simulink model "hexacopter_sim"  (R2024b)
settings: Solver=VariableStepAuto  StartTime=0  StopTime=100  FixedStep=0.1  RelTol=1e-3  EnableMultiTasking=on
values from neighbouring files (symbols this model uses):
  A = [zeros(4), eye(4); zeros(4),zeros(4)]    [hexacopter_par.m]
  b = 1.177*10^-5    (= 1.177e-05)    [hexacopter_par.m]
  B = [zeros(4) ... (first row only)    [hexacopter_par.m]
  C_obs = eye(8)    [hexacopter_par.m]
  d = 1.855*10^-7    (= 1.855e-07)    [hexacopter_par.m]
  fault_level = 0    [hexacopter_par.m]
  g = 9.81    [hexacopter_par.m]
  Ic = Ic + temp    [hexacopter_par.m]
  Ix = Ic(1,1)    [hexacopter_par.m]
  Iy = Ic(2,2)    [hexacopter_par.m]
  Iz = Ic(3,3)    [hexacopter_par.m]
  J_T = 1/2 *m_r* R_r^2    (= 0.0001)    [hexacopter_par.m]
  K_lqr = lqr(A', C_obs', Q, R)'    [hexacopter_par.m]
  K_phi = 0.03    [hexacopter_par.m]
  K_psi = 0.1    [hexacopter_par.m]
  K_theta = 0.03    [hexacopter_par.m]
  Kx = .1    (= 0.1)    [hexacopter_par.m]
  Ky = .1    (= 0.1)    [hexacopter_par.m]
  Kz = .1    (= 0.1)    [hexacopter_par.m]
  L = 0.275    [hexacopter_par.m]
  m = 2.5    [hexacopter_par.m]
  M_RB = [ m*eye(3) , zeros(3) ; zeros(3) , Ic ]    [hexacopter_par.m]
  motor_index = 3    [hexacopter_par.m]
  T_psinv = pinv(T)    [hexacopter_par.m]
libraries: slpidlib x19, simulink_extras x17, aerolibutil x2, matrix_library x2, vrlib x2, slctrl_smc x1
(part 1 of 3)
settings Model: Creator=The MathWorks, Inc.  LastModifiedBy=edtob
settings SolverCC: AlgebraicLoopSolver=TrustRegion
settings DataIOCC: LimitDataPoints=on  SaveFormat=Array  SaveOutput=off  SignalLogging=off  DSMLogging=off  SaveTime=off  ReturnWorkspaceOutputs=off
settings OptimizationCC: BlockReduction=off  BufferReuse=off  LifeSpan=inf
settings DebuggingCC: AlgebraicLoopMsg=none  ParameterPrecisionLossMsg=none  AllowSymbolicDim=off  PregeneratedLibrarySubsystemCodeDiagnostic=none  SFUnexpectedBacktrackingDiag=warning  SFNoUnconditionalDefaultTransitionDiag=warning  SFExecutionAtInitializationDiag=none  ArithmeticOperatorsInVariantConditions=warning
settings HardwareCC: ProdBitPerPointer=32  ProdBitPerSizeT=32  ProdBitPerPtrDiffT=32  ProdLargestAtomicFloat=None  ProdIntDivRoundTo=Undefined  ProdEndianess=Unspecified  ProdWordSize=32  ProdHWDeviceType=32-bit Generic
settings ModelReferenceCC: EnableRefExpFcnMdlSchedulingChecks=on  PropagateSignalLabelsOutOfModel=off
settings SFSimCC: SimUseLocalCustomCode=off  CustomCodeUndefinedFunction=UseInterfaceOnly
settings RTWCC: RTWUseLocalCustomCode=off  GPUComputeCapability=3.5  DLArmComputeVersion=19.05
settings CodeAppCC: StateflowObjectComments=on
settings GRTTargetCC: TargetLangStandard=C89/C90 (ANSI)
settings ConfigComp: CovMetricSettings=dw  CovSaveCumulativeToWorkspaceVar=on  CovSaveSingleToWorkspaceVar=on  CovExternalEMLEnable=off  CovSFcnEnable=off

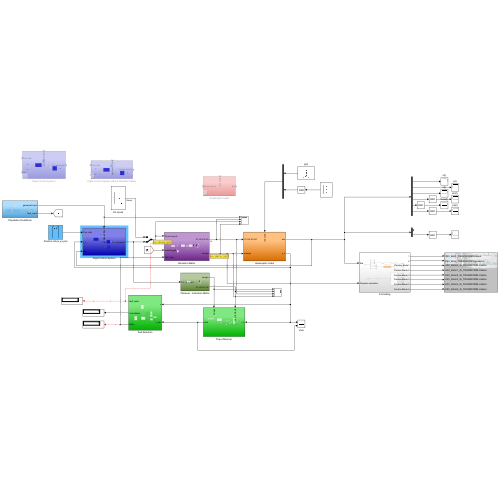
[thumbnail: Simulink's stored preview of the top-level diagram]
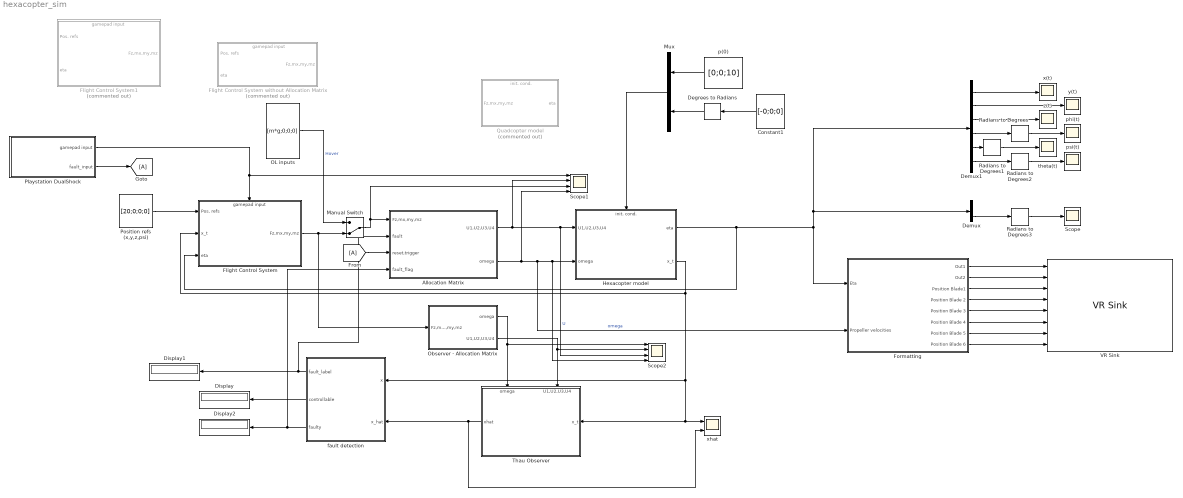
== system hexacopter_sim ==
  Allocation Matrix : Subsystem
  Constant1 : Constant  Value=[-0;0;0]  VectorParams1D=off
  Degrees to Radians : simulink_extras/Transformations/Degrees to Radians
  Demux : Demux  Outputs=2
  Demux1 : Demux  Outputs=6
  Display : Display
  Display1 : Display
  Display2 : Display
  Flight Control System : Subsystem
      settings: PortSchema="{\"entries\":[{\"content\":{\"sides\":[{\"content\":{\"connectorIds\":[\"In1\",\"In2\",\"In3\"]},\"type\":\"ConnectorPlacement.EquallySpacedRectSide\",\"uuid\":\"8ffec179-99fb-4b4c-a09d-a73fa0154dea\"},{\"content\":{\"connectorIds\":[\"Out1\"],\"side\":\"RIGHT\"},\"type\":\"ConnectorPlacement.EquallySpacedRectSide\",\"uuid\":\"b9ff487d-1da1-449a-81c9-f1838b0d3727\"},{\"content\":{\"connectorIds\":[\"In4\"],\"side\":\"TOP\"},\"type\":\"ConnectorPlacement.EquallySpacedRectSide\",\"uuid\":\"1948ac9a-8b1f-4a62-833b-18e2b106d39d\"}]},\"type\":\"ConnectorPlacement.EquallySpacedConnector\",\"uuid\":\"fea635f7-9753-4696-bad7-e2485c1b5acc\"}],\"packageUris\":[\"http://schema.mathworks.com/mf0/Connector/R2020b\"],\"version\":\"1.0\"}"
  Flight Control System without Allocation Matrix : Subsystem  Commented=on
      settings: PortSchema="{\"entries\":[{\"content\":{\"sides\":[{\"content\":{\"connectorIds\":[\"In1\",\"In2\"]},\"type\":\"ConnectorPlacement.EquallySpacedRectSide\",\"uuid\":\"8ffec179-99fb-4b4c-a09d-a73fa0154dea\"},{\"content\":{\"connectorIds\":[\"Out1\"],\"side\":\"RIGHT\"},\"type\":\"ConnectorPlacement.EquallySpacedRectSide\",\"uuid\":\"b9ff487d-1da1-449a-81c9-f1838b0d3727\"},{\"content\":{\"connectorIds\":[\"In3\"],\"side\":\"TOP\"},\"type\":\"ConnectorPlacement.EquallySpacedRectSide\",\"uuid\":\"1948ac9a-8b1f-4a62-833b-18e2b106d39d\"}]},\"type\":\"ConnectorPlacement.EquallySpacedConnector\",\"uuid\":\"fea635f7-9753-4696-bad7-e2485c1b5acc\"}],\"packageUris\":[\"http://schema.mathworks.com/mf0/Connector/R2020b\"],\"version\":\"1.0\"}"
  Flight Control System1 : Subsystem  Commented=on
      settings: PortSchema="{\"entries\":[{\"content\":{\"sides\":[{\"content\":{\"connectorIds\":[\"In1\",\"In2\"]},\"type\":\"ConnectorPlacement.EquallySpacedRectSide\",\"uuid\":\"8ffec179-99fb-4b4c-a09d-a73fa0154dea\"},{\"content\":{\"connectorIds\":[\"Out1\"],\"side\":\"RIGHT\"},\"type\":\"ConnectorPlacement.EquallySpacedRectSide\",\"uuid\":\"b9ff487d-1da1-449a-81c9-f1838b0d3727\"},{\"content\":{\"connectorIds\":[\"In3\"],\"side\":\"TOP\"},\"type\":\"ConnectorPlacement.EquallySpacedRectSide\",\"uuid\":\"1948ac9a-8b1f-4a62-833b-18e2b106d39d\"}]},\"type\":\"ConnectorPlacement.EquallySpacedConnector\",\"uuid\":\"fea635f7-9753-4696-bad7-e2485c1b5acc\"}],\"packageUris\":[\"http://schema.mathworks.com/mf0/Connector/R2020b\"],\"version\":\"1.0\"}"
  Formatting : Subsystem
  From : From
  Goto : Goto
  Hexacopter model : Subsystem
      settings: PortSchema="{\"entries\":[{\"content\":{\"sides\":[{\"content\":{\"connectorIds\":[\"In1\",\"In2\"]},\"type\":\"ConnectorPlacement.EquallySpacedRectSide\",\"uuid\":\"c5c2dfb8-9ff8-4aa4-96a6-7fa0d886c51f\"},{\"content\":{\"connectorIds\":[\"Out1\",\"Out2\"],\"side\":\"RIGHT\"},\"type\":\"ConnectorPlacement.EquallySpacedRectSide\",\"uuid\":\"2d7c7d5c-4ac5-4ebd-b09f-6a78733e851d\"},{\"content\":{\"connectorIds\":[\"In3\"],\"side\":\"TOP\"},\"type\":\"ConnectorPlacement.EquallySpacedRectSide\",\"uuid\":\"cf3a786d-06ed-46d4-985b-5c210afb13ec\"}]},\"type\":\"ConnectorPlacement.EquallySpacedConnector\",\"uuid\":\"cd57f0e6-7b9c-4392-8478-6e8af8e2560e\"}],\"packageUris\":[\"http://schema.mathworks.com/mf0/Connector/R2020b\"],\"version\":\"1.0\"}"
  Manual Switch : ManualSwitch  CurrentSetting=0
  Mux : Mux  Inputs=2
  OL inputs : Constant  Value=[m*g;0;0;0]  VectorParams1D=off
  Observer - Allocation Matrix : Subsystem
  Playstation DualShock : Subsystem
  Position refs (x,y,z,psi) : Constant  Value=[20;0;0;0]  VectorParams1D=off
  Quadcopter model : Subsystem  Commented=on
      settings: PortSchema="{\"entries\":[{\"content\":{\"sides\":[{\"content\":{\"connectorIds\":[\"In1\"]},\"type\":\"ConnectorPlacement.EquallySpacedRectSide\",\"uuid\":\"c5c2dfb8-9ff8-4aa4-96a6-7fa0d886c51f\"},{\"content\":{\"connectorIds\":[\"Out1\"],\"side\":\"RIGHT\"},\"type\":\"ConnectorPlacement.EquallySpacedRectSide\",\"uuid\":\"2d7c7d5c-4ac5-4ebd-b09f-6a78733e851d\"},{\"content\":{\"connectorIds\":[\"In2\"],\"side\":\"TOP\"},\"type\":\"ConnectorPlacement.EquallySpacedRectSide\",\"uuid\":\"cf3a786d-06ed-46d4-985b-5c210afb13ec\"}]},\"type\":\"ConnectorPlacement.EquallySpacedConnector\",\"uuid\":\"cd57f0e6-7b9c-4392-8478-6e8af8e2560e\"}],\"packageUris\":[\"http://schema.mathworks.com/mf0/Connector/R2020b\"],\"version\":\"1.0\"}"
  Radians to Degrees{,1..3} (4 alike) : simulink_extras/Transformations/Radians to Degrees
  Scope : Scope
  Scope1 : Scope  NumInputPorts=4
  Scope2 : Scope  NumInputPorts=4
  Thau Observer : Subsystem
      settings: PortSchema="{\"entries\":[{\"content\":{\"sides\":[{\"content\":{\"connectorIds\":[\"Out1\"]},\"type\":\"ConnectorPlacement.EquallySpacedRectSide\",\"uuid\":\"60a22802-45d1-4469-ac99-e897f8a02109\"},{\"content\":{\"connectorIds\":[\"In3\"],\"side\":\"RIGHT\"},\"type\":\"ConnectorPlacement.EquallySpacedRectSide\",\"uuid\":\"ce68a45a-4862-4479-bb8a-472f688a21a1\"},{\"content\":{\"connectorIds\":[\"In1\",\"In2\"],\"side\":\"TOP\"},\"type\":\"ConnectorPlacement.EquallySpacedRectSide\",\"uuid\":\"67c06515-e5f6-4d10-8c14-6a494d2e3ec4\"}]},\"type\":\"ConnectorPlacement.EquallySpacedConnector\",\"uuid\":\"39326fcb-b201-4ec9-b0d8-9908e3c571b8\"}],\"packageUris\":[\"http://schema.mathworks.com/mf0/Connector/R2020b\"],\"version\":\"1.0\"}"
  VR Sink : vrlib/VR Sink  InstantiateOnLoad=on  SampleTime=0.1  ViewEnable=on  RemoteChange=off  RemoteView=off  FieldsWritten=UAV_Body_TRANSFORM.rotation.4.1.1.double#UAV_Body_TRANSFORM.translation.3.1.1.double#UAV_Rotor4_ifs_TRANSFORM.rotation.4.1.1.double#UAV_Rotor1_ifs_TRANSFORM.rotation.4.1.1.double#UAV_Rotor5_ifs_TRANSFORM.rotation.4.1.1.double#UAV_Rotor3_ifs_TRANSFORM.rotation.4.1.1.double#UAV_Rotor2_ifs_TRANSFORM.rotation.4.1.1.double#UAV_Rotor6_ifs_TRANSFORM.rotation.4.1.1.double  WorldFileName=hexacopter_mesh_model\hexacopter_mesh_YfZu.x3d  AutoView=on  VideoDimensions=[]  AllowVariableSize=off
  fault detection : Subsystem
      settings: PortSchema="{\"entries\":[{\"content\":{\"sides\":[{\"content\":{},\"type\":\"ConnectorPlacement.EquallySpacedRectSide\",\"uuid\":\"736bf21b-0a48-4e94-ba78-b46e420ab8ca\"},{\"content\":{\"side\":\"RIGHT\"},\"type\":\"ConnectorPlacement.EquallySpacedRectSide\",\"uuid\":\"c3211a96-c27f-4c7f-93db-3db73ce054e6\"},{\"content\":{\"connectorIds\":[\"In1\",\"In2\"],\"side\":\"TOP\"},\"type\":\"ConnectorPlacement.EquallySpacedRectSide\",\"uuid\":\"5ce535da-2e21-4084-b8ee-f6acdfed52e0\"},{\"content\":{\"connectorIds\":[\"Out1\",\"Out2\",\"Out3\"],\"side\":\"BOTTOM\"},\"type\":\"ConnectorPlacement.EquallySpacedRectSide\",\"uuid\":\"102d30b0-f606-4160-8e28-2babae5d4ad1\"}]},\"type\":\"ConnectorPlacement.EquallySpacedConnector\",\"uuid\":\"782594a9-f93e-4bec-af89-e0648c48d7ab\"}],\"packageUris\":[\"http://schema.mathworks.com/mf0/Connector/R2020b\"],\"version\":\"1.0\"}"
  p(0) : Constant  Value=[0;0;10]  VectorParams1D=off
  phi(t) : Scope
  psi(t) : Scope
  theta(t) : Scope
  x(t) : Scope
  xhat : Scope  NumInputPorts=2
  y(t) : Scope
  z(t) : Scope
  wires:
  Radians to Degrees2/1 -> psi(t)/1
  Demux1/6 -> Radians to Degrees2/1
  p(0)/1 -> Mux/1
  Demux1/4 -> Radians to Degrees/1
  Degrees to Radians/1 -> Mux/2
  Demux1/3 -> z(t)/1
  Demux1/2 -> y(t)/1
  Radians to Degrees/1 -> phi(t)/1
  Position refs (x,y,z,psi)/1 -> Flight Control System/1(Pos. refs)
  Constant1/1 -> Degrees to Radians/1
  Demux1/1 -> x(t)/1
  Radians to Degrees1/1 -> theta(t)/1
  Mux/1 -> Hexacopter model/3(init. cond.)
  Demux1/5 -> Radians to Degrees1/1
  OL inputs/1 -> Manual Switch/1  "Hover"
  Playstation DualShock/1(gamepad input) -> Flight Control System/4(gamepad input), Scope1/1
  Formatting/1(Out1) -> VR Sink/1
  Formatting/2(Out2) -> VR Sink/2
  Formatting/3(Position Blade1) -> VR Sink/3
  Formatting/4(Position Blade 2) -> VR Sink/4
  Formatting/5(Position Blade 3) -> VR Sink/5
  Formatting/6(Position Blade 4) -> VR Sink/6
  Formatting/7(Position Blade 5) -> VR Sink/7
  Formatting/8(Position Blade 6) -> VR Sink/8
  Allocation Matrix/2(omega) -> Scope1/4, Formatting/2(Propeller velocities), Scope2/4, Hexacopter model/2(omega)  "omega"
  fault detection/2(controllable) -> Display/1
  Thau Observer/1(xhat) -> xhat/2, fault detection/2(x_hat)
  Manual Switch/1 -> Scope1/3, Allocation Matrix/1(Fz,mx,my,mz)
  fault detection/1(fault_label) -> Allocation Matrix/2(fault), Display1/1
  Hexacopter model/2(x_t) -> fault detection/1(x), Thau Observer/3(x_t), xhat/1, Flight Control System/2(x_t)
  Playstation DualShock/2(fault_input) -> Goto/1
  From/1 -> Allocation Matrix/3(reset,trigger)
  Hexacopter model/1(eta) -> Flight Control System/3(eta), Formatting/1(Eta), Demux/1, Demux1/1
  Demux/2 -> Radians to Degrees3/1
  Radians to Degrees3/1 -> Scope/1
  Observer - Allocation Matrix/1(omega) -> Thau Observer/1(omega), Scope2/1
  Observer - Allocation Matrix/2(U1,U2,U3,U4) -> Thau Observer/2(U1,U2,U3,U4), Scope2/2
  Allocation Matrix/1(U1,U2,U3,U4) -> Scope2/3, Hexacopter model/1(U1,U2,U3,U4), Scope1/2  "U"
  fault detection/3(faulty) -> Allocation Matrix/4(fault_flag), Display2/1
  Flight Control System/1(Fz,mx,my,mz) -> Observer - Allocation Matrix/1(Fz,mx,my,mz), Manual Switch/2

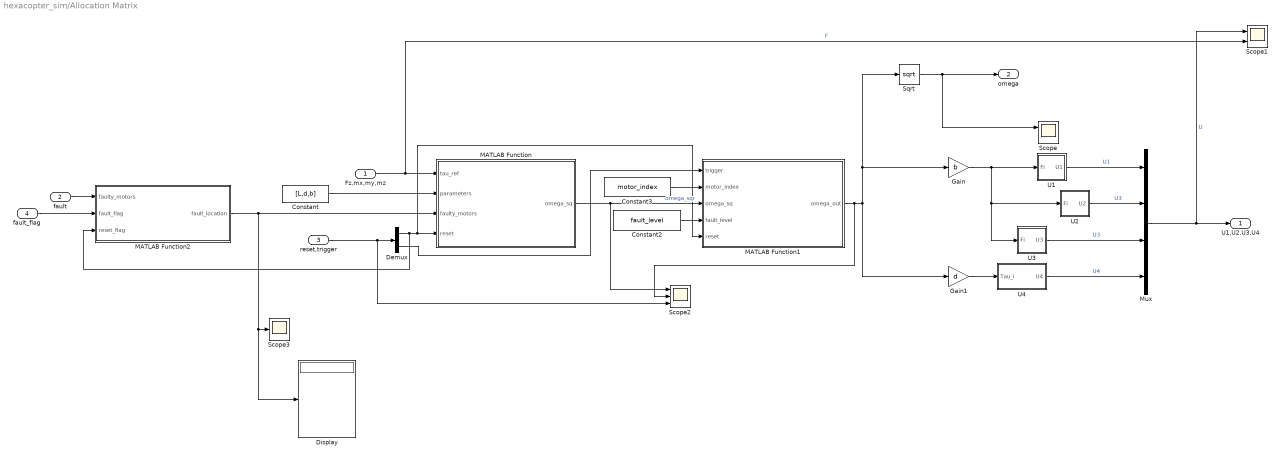
== system hexacopter_sim/Allocation Matrix ==
  Fz,mx,my,mz : Inport
  fault : Inport  Port=2
  reset,trigger : Inport  Port=3
  fault_flag : Inport  Port=4
  Constant : Constant  Value=[L,d,b]
  Constant2 : Constant  Value=fault_level
  Constant3 : Constant  Value=motor_index
  Demux : Demux  Outputs=2
  Display : Display
  Gain : Gain  Gain=b
  Gain1 : Gain  Gain=d
  MATLAB Function : MATLAB Function  TreatAsAtomicUnit=on
  MATLAB Function1 : MATLAB Function  TreatAsAtomicUnit=on
  MATLAB Function2 : MATLAB Function  TreatAsAtomicUnit=on
  Mux : Mux
  Scope : Scope  NumInputPorts=2
  Scope1 : Scope  NumInputPorts=2
  Scope2 : Scope  NumInputPorts=3
  Scope3 : Scope
  Sqrt : Sqrt
  U1 : Subsystem
  U2 : Subsystem
  U3 : Subsystem
  U4 : Subsystem
  U1,U2,U3,U4 : Outport
  omega : Outport  Port=2
  wires:
  fault/1 -> MATLAB Function2/1(faulty_motors)
  Fz,mx,my,mz/1 -> Scope1/2, MATLAB Function/1(tau_ref)  "F"
  Gain/1 -> U2/1(Fi), U3/1(Fi), U1/1(Fi)
  U1/1(U1) -> Mux/1  "U1"
  Gain1/1 -> U4/1(Tau_i)
  U4/1(U4) -> Mux/4  "U4"
  Mux/1 -> Scope1/1, U1,U2,U3,U4/1  "U"
  Sqrt/1 -> Scope/1, omega/1
  Constant/1 -> MATLAB Function/2(parameters)
  MATLAB Function/1(omega_sq) -> Scope2/1, MATLAB Function1/3(omega_sq)  "omega_sqr"
  MATLAB Function1/1(omega_out) -> Scope2/2, Gain1/1, Sqrt/1, Gain/1
  Constant2/1 -> MATLAB Function1/4(fault_level)
  Constant3/1 -> MATLAB Function1/2(motor_index)
  reset,trigger/1 -> Scope2/3, Demux/1
  Demux/1 -> MATLAB Function2/3(reset_flag), MATLAB Function1/5(reset), MATLAB Function/4(reset)
  Demux/2 -> MATLAB Function1/1(trigger)
  U3/1(U3) -> Mux/3  "U3"
  U2/1(U2) -> Mux/2  "U3"
  MATLAB Function2/1(fault_location) -> Display/1, Scope3/1, MATLAB Function/3(faulty_motors)
  fault_flag/1 -> MATLAB Function2/2(fault_flag)

== system hexacopter_sim/Flight Control System ==
  Pos. refs : Inport
  x_t : Inport  Port=2
  eta : Inport  Port=3
  gamepad input : Inport  Port=4
  Gain : Gain  Gain=10000
  Inner-loop PID controllers : Subsystem
  Inner-loop PID controllers1 : Subsystem  Commented=on
  Manual Switch : ManualSwitch
  Manual Switch1 : ManualSwitch
  Manual Switch2 : ManualSwitch
  Outer loop position control : Subsystem
  desired z,phictheta,psi : Constant  Value=[-10;0;0;0]  VectorParams1D=off
  Fz,mx,my,mz : Outport
  wires:
  Manual Switch/1 -> Inner-loop PID controllers1/1(desired z,phictheta,psi), Inner-loop PID controllers/1(desired z,phictheta,psi)
  eta/1 -> Outer loop position control/2(eta), Inner-loop PID controllers1/3(eta), Inner-loop PID controllers/2(eta)
  Pos. refs/1 -> Outer loop position control/1(Pos. refs)
  Outer loop position control/1(desired z,phi,theta,psi) -> Manual Switch/2
  desired z,phictheta,psi/1 -> Manual Switch1/2
  Manual Switch1/1 -> Manual Switch/1
  gamepad input/1 -> Manual Switch1/1
  Inner-loop PID controllers1/1(Fz,mx,my,mz) -> Manual Switch2/2
  Manual Switch2/1 -> Fz,mx,my,mz/1
  x_t/1 -> Inner-loop PID controllers1/2(x_t)
  Inner-loop PID controllers/1(Fz,mx,my,mz) -> Gain/1
  Gain/1 -> Manual Switch2/1

== system hexacopter_sim/Flight Control System without Allocation Matrix ==
  Pos. refs : Inport
  eta : Inport  Port=2
  gamepad input : Inport  Port=3
  Inner-loop PID controllers : Subsystem
  Manual Switch : ManualSwitch
  Manual Switch1 : ManualSwitch
  Outer loop position control : Subsystem
  desired z,phictheta,psi : Constant  Value=[-10;20;0;0]  VectorParams1D=off
  Fz,mx,my,mz : Outport
  wires:
  Inner-loop PID controllers/1(Fz,mx,my,mz) -> Fz,mx,my,mz/1
  Manual Switch/1 -> Inner-loop PID controllers/1(desired z,phictheta,psi)
  eta/1 -> Outer loop position control/2(eta), Inner-loop PID controllers/2(eta)
  Pos. refs/1 -> Outer loop position control/1(Pos. refs)
  Outer loop position control/1(desired z,phi,theta,psi) -> Manual Switch/2
  desired z,phictheta,psi/1 -> Manual Switch1/2
  Manual Switch1/1 -> Manual Switch/1
  gamepad input/1 -> Manual Switch1/1

== system hexacopter_sim/Flight Control System1 ==
  Pos. refs : Inport
  eta : Inport  Port=2
  gamepad input : Inport  Port=3
  Inner-loop PID controllers : Subsystem
  Manual Switch : ManualSwitch
  Manual Switch1 : ManualSwitch
  Outer loop position control : Subsystem
  desired z,phictheta,psi : Constant  Value=[-10;0;0;0]  VectorParams1D=off
  Fz,mx,my,mz : Outport
  wires:
  gamepad input/1 -> Manual Switch1/1
  Manual Switch1/1 -> Manual Switch/1
  desired z,phictheta,psi/1 -> Manual Switch1/2
  Outer loop position control/1(desired z,phi,theta,psi) -> Manual Switch/2
  Pos. refs/1 -> Outer loop position control/1(Pos. refs)
  eta/1 -> Inner-loop PID controllers/2(eta), Outer loop position control/2(eta)
  Manual Switch/1 -> Inner-loop PID controllers/1(desired z,phictheta,psi)
  Inner-loop PID controllers/1(Fz,mx,my,mz) -> Fz,mx,my,mz/1

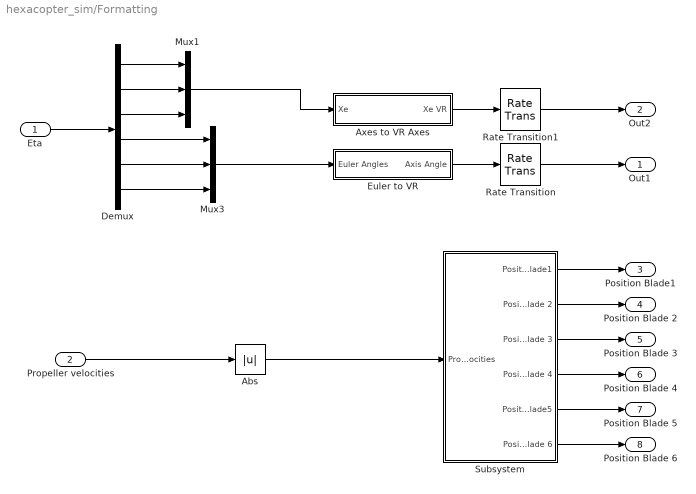
== system hexacopter_sim/Formatting ==
  Eta : Inport
  Propeller velocities : Inport  Port=2
  Abs : Abs  SaturateOnIntegerOverflow=off
  Axes to VR Axes : Subsystem
  Demux : Demux  Outputs=6
  Euler to VR : Subsystem
  Mux1 : Mux  Inputs=3
  Mux3 : Mux  Inputs=3
  Rate Transition : RateTransition
  Rate Transition1 : RateTransition
  Subsystem : Subsystem
  Out1 : Outport
  Out2 : Outport  Port=2
  Position Blade1 : Outport  Port=3
  Position Blade 2 : Outport  Port=4
  Position Blade 3 : Outport  Port=5
  Position Blade 4 : Outport  Port=6
  Position Blade 5 : Outport  Port=7
  Position Blade 6 : Outport  Port=8
  wires:
  Subsystem/3(Position Blade 3) -> Position Blade 3/1
  Subsystem/1(Position Blade1) -> Position Blade1/1
  Mux3/1 -> Euler to VR/1(Euler Angles)
  Subsystem/2(Position Blade 2) -> Position Blade 2/1
  Euler to VR/1(Axis Angle) -> Rate Transition/1
  Axes to VR Axes/1(Xe VR) -> Rate Transition1/1
  Rate Transition1/1 -> Out2/1
  Mux1/1 -> Axes to VR Axes/1(Xe)
  Rate Transition/1 -> Out1/1
  Subsystem/4(Position Blade 4) -> Position Blade 4/1
  Demux/2 -> Mux1/2
  Demux/5 -> Mux3/2
  Demux/3 -> Mux1/3
  Eta/1 -> Demux/1
  Demux/1 -> Mux1/1
  Demux/4 -> Mux3/1
  Demux/6 -> Mux3/3
  Subsystem/5(Position Blade5) -> Position Blade 5/1
  Subsystem/6(Position Blade 6) -> Position Blade 6/1
  Propeller velocities/1 -> Abs/1
  Abs/1 -> Subsystem/1(Propeller velocities)

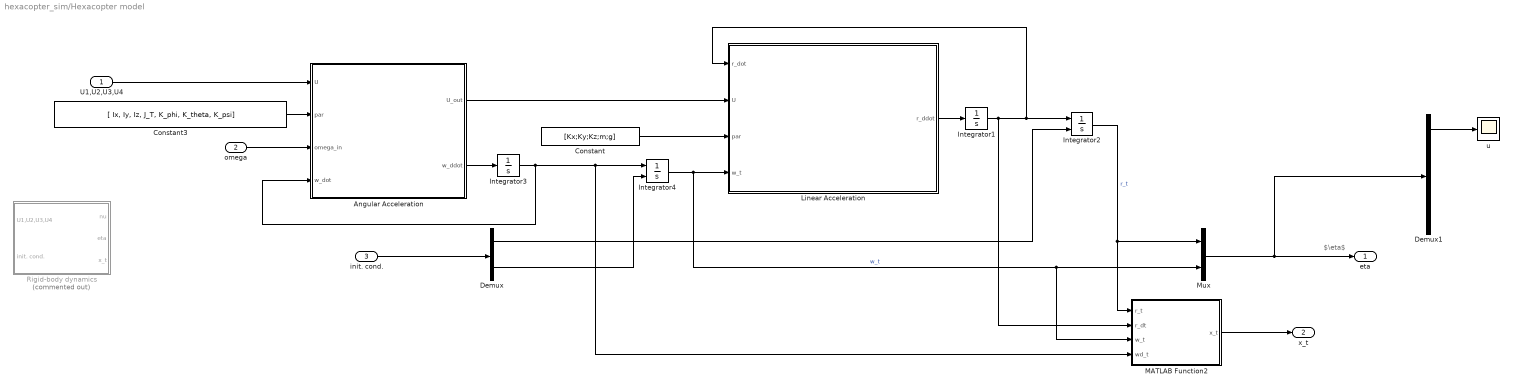
== system hexacopter_sim/Hexacopter model ==
  note: $\eta$
  U1,U2,U3,U4 : Inport
  omega : Inport  Port=2
  init. cond. : Inport  Port=3
  "Angular Acceleration " : MATLAB Function  TreatAsAtomicUnit=on
  Constant : Constant  Value=[Kx;Ky;Kz;m;g]
  Constant3 : Constant  Value=[ Ix, Iy, Iz, J_T, K_phi, K_theta, K_psi]
  Demux : Demux  Outputs=2
  Demux1 : Demux  Outputs=6
  Integrator1 : Integrator  InitialCondition=[0;0;0]
  Integrator2 : Integrator  InitialConditionSource=external
  Integrator3 : Integrator  InitialCondition=[0;0;0]
  Integrator4 : Integrator  InitialConditionSource=external
  Linear Acceleration : MATLAB Function  TreatAsAtomicUnit=on
  MATLAB Function2 : MATLAB Function  TreatAsAtomicUnit=on
  Mux : Mux  Inputs=2
  Rigid-body dynamics : Subsystem  Commented=on
  u : Scope
  eta : Outport
  x_t : Outport  Port=2
  wires:
  Demux1/1 -> u/1
  Constant/1 -> Linear Acceleration/3(par)
  Demux/1 -> Integrator2/2
  Mux/1 -> Demux1/1, eta/1
  Integrator4/1 -> MATLAB Function2/3(w_t), Mux/2, Linear Acceleration/4(w_t)  "w_t"
  Demux/2 -> Integrator4/2
  MATLAB Function2/1(x_t) -> x_t/1
  init. cond./1 -> Demux/1
  Integrator3/1 -> MATLAB Function2/4(wd_t), Integrator4/1, "Angular Acceleration "/4(w_dot)
  "Angular Acceleration "/2(w_ddot) -> Integrator3/1
  Linear Acceleration/1(r_ddot) -> Integrator1/1
  Integrator2/1 -> MATLAB Function2/1(r_t), Mux/1  "r_t"
  U1,U2,U3,U4/1 -> "Angular Acceleration "/1(U)
  Constant3/1 -> "Angular Acceleration "/2(par)
  "Angular Acceleration "/1(U_out) -> Linear Acceleration/2(U)
  Integrator1/1 -> MATLAB Function2/2(r_dt), Linear Acceleration/1(r_dot), Integrator2/1
  omega/1 -> "Angular Acceleration "/3(omega_in)

== system hexacopter_sim/Observer - Allocation Matrix ==
  Fz,mx,my,mz : Inport
  Constant : Constant  Value=T_psinv
  Gain : Gain  Gain=b
  Gain1 : Gain  Gain=d
  MATLAB Function : MATLAB Function  TreatAsAtomicUnit=on
  Mux : Mux
  Sqrt : Sqrt
  U1 : Subsystem
  U2 : Subsystem
  U3 : Subsystem
  U4 : Subsystem
  omega : Outport
  U1,U2,U3,U4 : Outport  Port=2
  wires:
  MATLAB Function/1(omega_sq) -> Gain1/1, Gain/1, Sqrt/1  "omega_sqr"
  Fz,mx,my,mz/1 -> MATLAB Function/1(tau_ref)
  Sqrt/1 -> omega/1
  Constant/1 -> MATLAB Function/2(T_psinv)
  U3/1(U3) -> Mux/3  "U3"
  U2/1(U2) -> Mux/2  "U3"
  Gain/1 -> U2/1(Fi), U3/1(Fi), U1/1(Fi)
  Gain1/1 -> U4/1(Tau_i)
  U1/1(U1) -> Mux/1  "U1"
  Mux/1 -> U1,U2,U3,U4/1  "U"
  U4/1(U4) -> Mux/4  "U4"

== system hexacopter_sim/Playstation DualShock ==
  Formatting : Subsystem
  Gamepad : vrlib/Joystick Input  joyid=1  adjustports=on  forcefeed=off
  Mux : Mux  Inputs=2
  Scope : Scope
  gamepad input : Outport
  fault_input : Outport  Port=2
  wires:
  Formatting/1(gamepad input) -> gamepad input/1
  Gamepad/2 -> Formatting/2(Buttons)
  Gamepad/1 -> Scope/1, Formatting/1(Axes)
  Gamepad/3 -> Formatting/3(Point of View)
  Formatting/3(trigger) -> Mux/2
  Formatting/2(reset) -> Mux/1
  Mux/1 -> fault_input/1

== system hexacopter_sim/Quadcopter model ==
  note: $\eta$
  Fz,mx,my,mz : Inport
  init. cond. : Inport  Port=2
  Demux : Demux
  Demux1 : Demux  Outputs=6
  Ground : Ground
  Ground1 : Ground
  Kinematics : Subsystem
  Mux1 : Mux  Inputs=6
  Rigid-body dynamics : Subsystem
  gravity : Subsystem
  u : Scope
  eta : Outport
  wires:
  Ground1/1 -> Mux1/1
  Kinematics/1(R_be) -> gravity/1(R_be)
  Kinematics/2(eta) -> eta/1
  gravity/1(tau_g) -> Rigid-body dynamics/1(tau_g)
  Mux1/1 -> Rigid-body dynamics/2(tau_p)
  Rigid-body dynamics/1(nu) -> Demux1/1, Kinematics/1(nu)
  init. cond./1 -> Kinematics/2(init. cond.)
  Demux1/1 -> u/1
  Fz,mx,my,mz/1 -> Demux/1
  Demux/2 -> Mux1/4
  Demux/3 -> Mux1/5
  Demux/4 -> Mux1/6
  Ground/1 -> Mux1/2
  Demux/1 -> Mux1/3

== system hexacopter_sim/Thau Observer ==
  omega : Inport
  U1,U2,U3,U4 : Inport  Port=2
  x_t : Inport  Port=3
  Constant : Constant  Value=[Ix,Iy,Iz, J_T,g]  VectorParams1D=off
  Gain : Gain  Gain=A  Multiplication=Matrix(K*u)
  Gain1 : Gain  Gain=B  Multiplication=Matrix(K*u)
  Gain2 : Gain  Gain=C_obs  Multiplication=Matrix(K*u)
  Gain3 : Gain  Gain=K_lqr  Multiplication=Matrix(K*u)
  Gain4 : Gain  Gain=C_obs  Multiplication=Matrix(K*u)
  Integrator : Integrator  InitialCondition=[0;0;0;0;0;0;10;0]
  MATLAB Function : MATLAB Function  TreatAsAtomicUnit=on
  Sum : Sum  Inputs=|++++
  Sum1 : Sum  Inputs=|+-
  U2,U3,U4,U1 : Selector  InputPortWidth=4  IndexOptions=Index vector (dialog)  Indices=[2 3 4 1]  OutputSizes=1
  xhat : Outport
  wires:
  Constant/1 -> MATLAB Function/1(misc)
  x_t/1 -> Gain4/1
  Integrator/1 -> MATLAB Function/3(xhat), Gain2/1, Gain/1, xhat/1  "xhat"
  U1,U2,U3,U4/1 -> U2,U3,U4,U1/1
  omega/1 -> MATLAB Function/2(omega_in)
  U2,U3,U4,U1/1 -> Gain1/1
  MATLAB Function/1(hx) -> Sum/1
  Gain1/1 -> Sum/2
  Sum/1 -> Integrator/1
  Gain3/1 -> Sum/3
  Gain/1 -> Sum/4
  Gain4/1 -> Sum1/1  "y_t"
  Gain2/1 -> Sum1/2  "yhat"
  Sum1/1 -> Gain3/1

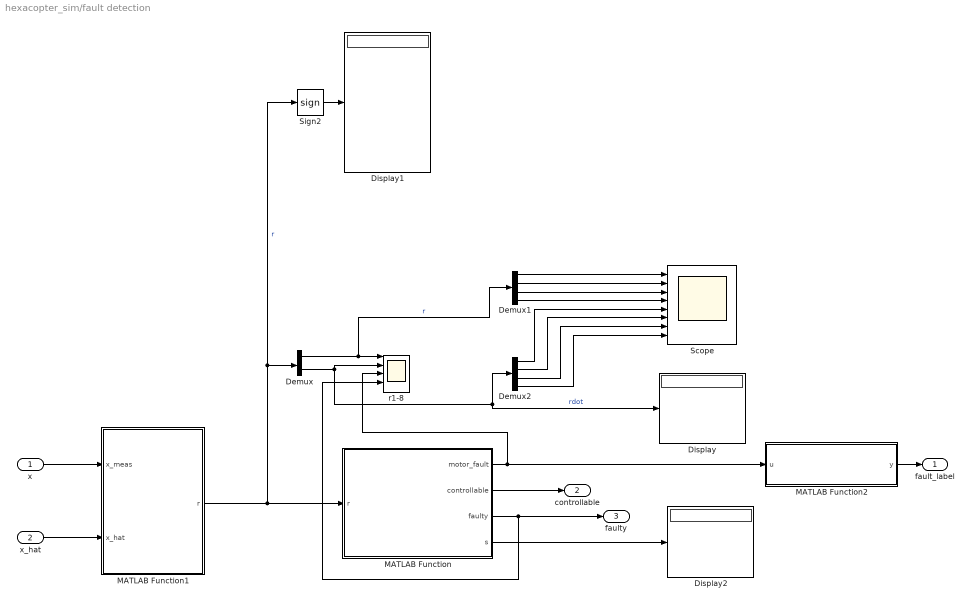
== system hexacopter_sim/fault detection ==
  x : Inport
  x_hat : Inport  Port=2
  Demux : Demux  Outputs=2
  Demux1 : Demux
  Demux2 : Demux
  Display : Display
  Display1 : Display
  Display2 : Display
  MATLAB Function : MATLAB Function  TreatAsAtomicUnit=on
  MATLAB Function1 : MATLAB Function  TreatAsAtomicUnit=on
  MATLAB Function2 : MATLAB Function  TreatAsAtomicUnit=on
  Scope : Scope  NumInputPorts=8
  Sign2 : Signum
  r1-8 : Scope  NumInputPorts=5
  fault_label : Outport
  controllable : Outport  Port=2
  faulty : Outport  Port=3
  wires:
  x/1 -> MATLAB Function1/1(x_meas)
  x_hat/1 -> MATLAB Function1/2(x_hat)
  MATLAB Function/2(controllable) -> controllable/1
  MATLAB Function1/1(r) -> Demux/1, Sign2/1, MATLAB Function/1(r)  "r"
  Demux/1 -> Demux1/1, r1-8/1  "r"
  Demux/2 -> Demux2/1, Display/1, r1-8/2  "rdot"
  MATLAB Function/3(faulty) -> faulty/1, r1-8/4
  Demux1/1 -> Scope/1
  Demux1/2 -> Scope/2
  Demux1/3 -> Scope/3
  Demux1/4 -> Scope/4
  Demux2/1 -> Scope/5
  Demux2/2 -> Scope/6
  Demux2/3 -> Scope/7
  Demux2/4 -> Scope/8
  Sign2/1 -> Display1/1
  MATLAB Function/4(s) -> Display2/1
  MATLAB Function/1(motor_fault) -> MATLAB Function2/1(u), r1-8/3
  MATLAB Function2/1(y) -> fault_label/1

== system hexacopter_sim/Allocation Matrix/U1 ==
  Fi : Inport
  Demux : Demux  Outputs=6
  Sum of Elements : Sum  Inputs=++++++
  U1 : Outport
  wires:
  Fi/1 -> Demux/1
  Demux/2 -> Sum of Elements/2  "F2"
  Demux/1 -> Sum of Elements/1  "F1"
  Demux/3 -> Sum of Elements/3  "F3"
  Demux/4 -> Sum of Elements/4  "F4"
  Demux/5 -> Sum of Elements/5  "F5"
  Demux/6 -> Sum of Elements/6  "F6"
  Sum of Elements/1 -> U1/1

== system hexacopter_sim/Allocation Matrix/U2 ==
  Fi : Inport
  Demux : Demux  Outputs=6
  Gain : Gain  Gain=1/2
  Gain1 : Gain  Gain=L
  Sum : Sum  Inputs=|-+
  Sum of Elements : Sum  Inputs=-++-
  Sum1 : Sum  Inputs=|++
  U2 : Outport
  wires:
  Fi/1 -> Demux/1
  Demux/1 -> Sum/1  "F1"
  Demux/6 -> Sum of Elements/4  "F6"
  Demux/5 -> Sum of Elements/3  "F5"
  Sum of Elements/1 -> Gain/1
  Sum/1 -> Sum1/1
  Gain/1 -> Sum1/2
  Sum1/1 -> Gain1/1
  Gain1/1 -> U2/1
  Demux/2 -> Sum of Elements/1  "F2"
  Demux/4 -> Sum/2  "F4"
  Demux/3 -> Sum of Elements/2  "F3"

== system hexacopter_sim/Allocation Matrix/U3 ==
  Fi : Inport
  Demux : Demux  Outputs=6
  Gain : Gain  Gain=L/2*sqrt(3)
  Sum of Elements : Sum  Inputs=++--
  Terminator : Terminator
  Terminator1 : Terminator
  U3 : Outport
  wires:
  Sum of Elements/1 -> Gain/1
  Demux/5 -> Sum of Elements/3  "F5"
  Demux/6 -> Sum of Elements/4  "F6"
  Fi/1 -> Demux/1
  Demux/1 -> Terminator/1  "F1"
  Demux/2 -> Sum of Elements/1  "F2"
  Gain/1 -> U3/1
  Demux/4 -> Terminator1/1  "F4"
  Demux/3 -> Sum of Elements/2  "F3"

== system hexacopter_sim/Allocation Matrix/U4 ==
  Tau_i : Inport
  Demux : Demux  Outputs=6
  Sum of Elements : Sum  Inputs=-+--++
  U4 : Outport
  wires:
  Tau_i/1 -> Demux/1
  Sum of Elements/1 -> U4/1
  Demux/1 -> Sum of Elements/1  "Tau_1"
  Demux/2 -> Sum of Elements/2  "Tau_2"
  Demux/3 -> Sum of Elements/3  "Tau_3"
  Demux/4 -> Sum of Elements/4  "Tau_4"
  Demux/5 -> Sum of Elements/5  "Tau_5"
  Demux/6 -> Sum of Elements/6  "Tau_6"

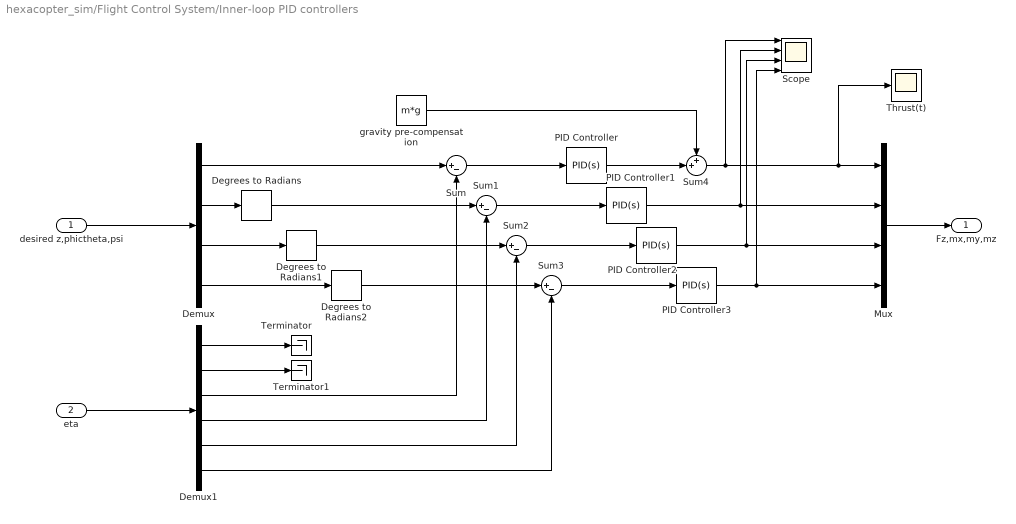
== system hexacopter_sim/Flight Control System/Inner-loop PID controllers ==
  desired z,phictheta,psi : Inport
  eta : Inport  Port=2
  Degrees to Radians : simulink_extras/Transformations/Degrees to Radians
  Degrees to Radians1 : simulink_extras/Transformations/Degrees to Radians
  Degrees to Radians2 : simulink_extras/Transformations/Degrees to Radians
  Demux : Demux
  Demux1 : Demux  Outputs=6
  Mux : Mux
  PID Controller : slpidlib/PID Controller  Controller=PID  Form=Parallel  TimeDomain=Continuous-time  UseExternalTs=off  SampleTime=-1  IntegratorMethod=Forward Euler  FilterMethod=Forward Euler  ControllerParametersSource=internal  P=0.00835190565465849  I=7.76570674719384e-05  UseKiTs=off  D=0.156681263051577  UseExternalDerivativeSource=off  N=0.259802011561812  UseFilter=on  TunerSelectOption=Transfer Function Based (PID Tuner App)  InitialConditionSource=internal  InitialConditionForIntegrator=0  InitialConditionForFilter=0  DifferentiatorICPrevScaledInput=0  ExternalReset=none  TrackingMode=off  Kt=1  LimitOutput=off  SatLimitsSource=internal  UpperSaturationLimit=inf  LowerSaturationLimit=-inf  LinearizeAsGain=on  AntiWindupMode=none  Kb=1  LimitIntegrator=off  UpperIntegratorSaturationLimit=inf  LowerIntegratorSaturationLimit=-inf  POutMin=[]  POutMax=[]  IOutMin=[]  IOutMax=[]  DOutMin=[]  DOutMax=[]  NOutMin=[]  NOutMax=[]  SumOutMin=[]  SumOutMax=[]  SaturationOutMin=[]  SaturationOutMax=[]  PParamMin=[]  PParamMax=[]  IParamMin=[]  IParamMax=[]  DParamMin=[]  DParamMax=[]  NParamMin=[]  NParamMax=[]  KbParamMin=[]  KbParamMax=[]  KtParamMin=[]  KtParamMax=[]  KbOutMin=[]  KbOutMax=[]  KtOutMin=[]  KtOutMax=[]  IntegratorOutMin=[]  IntegratorOutMax=[]  FilterOutMin=[]  FilterOutMax=[]  SumI1OutMin=[]  SumI1OutMax=[]  SumI2OutMin=[]  SumI2OutMax=[]  SumI3OutMin=[]  SumI3OutMax=[]  SumI4OutMin=[]  SumI4OutMax=[]  SumDOutMin=[]  SumDOutMax=[]  DifferentiatorOutMin=[]  DifferentiatorOutMax=[]  FilterDiffOutCoefMin=[]  FilterDiffOutCoefMax=[]  ReciprocalOutMin=[]  ReciprocalOutMax=[]  SumDenOutMin=[]  SumDenOutMax=[]  SumNumOutMin=[]  SumNumOutMax=[]  DivideOutMin=[]  DivideOutMax=[]  UdiffTsProdOutMin=[]  UdiffTsProdOutMax=[]  NTsProdOutMin=[]  NTsProdOutMax=[]  UintegralTsProdOutMin=[]  UintegralTsProdOutMax=[]  UngainTsProdOutMin=[]  UngainTsProdOutMax=[]  ClampingZeroOutDataTypeStr=Inherit: Inherit via back propagation  ClampingZeroOutMin=[]  ClampingZeroOutMax=[]  FilterDenConstantOutDataTypeStr=Inherit: Inherit via back propagation  FilterDenConstantOutMin=[]  FilterDenConstantOutMax=[]  PCopyOutDataTypeStr=Inherit: Inherit via back propagation  PCopyOutMin=[]  PCopyOutMax=[]  NCopyOutDataTypeStr=Inherit: Inherit via back propagation  NCopyOutMin=[]  NCopyOutMax=[]  IntegratorContinuousStateAttributes=''  IntegratorStateMustResolveToSignalObject=off  IntegratorRTWStateStorageClass=Auto  FilterContinuousStateAttributes=''  FilterStateMustResolveToSignalObject=off  FilterRTWStateStorageClass=Auto  ParallelPVariant=InternalParameters  IdealPVariant=Disabled  IVariant=InternalParameters  DVariant=InternalParameters  IntegratorVariant=Continuous  SatVariant=Disabled  AWVariant=Passthrough  PCopyVariant=Disabled  TRVariant=Disabled  FdbkBlocksVariant=Forward  IdealPFdbkVariant=Disabled  SatFdbkVariant=Disabled  DerivativeFilterVariant=ContFilter  NVariant=InternalParameters  NCopyVariant=Disabled  FilterICVariant=InternalICsFilter  IntegratorICVariant=InternalICs  ExternalResetVariant=Disabled  TRSumVariant=Passthrough  SumFdbkVariant=Disabled  SumVariant=Sum_PID  TsampFilterVariant=InternalTs  TsampNgainVariant=Passthrough  TsampIntegralVariant=Disabled_SignalSpec  ExternalSaturationOutDataTypeStr=Inherit: Same as second input  DerivativeSourceVariant=ErrorSignal  PreIntVariant=InternalPreInt
  PID Controller1 : slpidlib/PID Controller  Controller=PID  Form=Parallel  TimeDomain=Continuous-time  UseExternalTs=off  SampleTime=-1  IntegratorMethod=Forward Euler  FilterMethod=Forward Euler  ControllerParametersSource=internal  P=0.207161479002829  I=0.156816518259524  UseKiTs=off  D=0.0473265688761706  UseExternalDerivativeSource=off  N=21.4472408149803  UseFilter=on  TunerSelectOption=Transfer Function Based (PID Tuner App)  InitialConditionSource=internal  InitialConditionForIntegrator=0  InitialConditionForFilter=0  DifferentiatorICPrevScaledInput=0  ExternalReset=none  TrackingMode=off  Kt=1  LimitOutput=off  SatLimitsSource=internal  UpperSaturationLimit=inf  LowerSaturationLimit=-inf  LinearizeAsGain=on  AntiWindupMode=none  Kb=1  LimitIntegrator=off  UpperIntegratorSaturationLimit=inf  LowerIntegratorSaturationLimit=-inf  POutMin=[]  POutMax=[]  IOutMin=[]  IOutMax=[]  DOutMin=[]  DOutMax=[]  NOutMin=[]  NOutMax=[]  SumOutMin=[]  SumOutMax=[]  SaturationOutMin=[]  SaturationOutMax=[]  PParamMin=[]  PParamMax=[]  IParamMin=[]  IParamMax=[]  DParamMin=[]  DParamMax=[]  NParamMin=[]  NParamMax=[]  KbParamMin=[]  KbParamMax=[]  KtParamMin=[]  KtParamMax=[]  KbOutMin=[]  KbOutMax=[]  KtOutMin=[]  KtOutMax=[]  IntegratorOutMin=[]  IntegratorOutMax=[]  FilterOutMin=[]  FilterOutMax=[]  SumI1OutMin=[]  SumI1OutMax=[]  SumI2OutMin=[]  SumI2OutMax=[]  SumI3OutMin=[]  SumI3OutMax=[]  SumI4OutMin=[]  SumI4OutMax=[]  SumDOutMin=[]  SumDOutMax=[]  DifferentiatorOutMin=[]  DifferentiatorOutMax=[]  FilterDiffOutCoefMin=[]  FilterDiffOutCoefMax=[]  ReciprocalOutMin=[]  ReciprocalOutMax=[]  SumDenOutMin=[]  SumDenOutMax=[]  SumNumOutMin=[]  SumNumOutMax=[]  DivideOutMin=[]  DivideOutMax=[]  UdiffTsProdOutMin=[]  UdiffTsProdOutMax=[]  NTsProdOutMin=[]  NTsProdOutMax=[]  UintegralTsProdOutMin=[]  UintegralTsProdOutMax=[]  UngainTsProdOutMin=[]  UngainTsProdOutMax=[]  ClampingZeroOutDataTypeStr=Inherit: Inherit via back propagation  ClampingZeroOutMin=[]  ClampingZeroOutMax=[]  FilterDenConstantOutDataTypeStr=Inherit: Inherit via back propagation  FilterDenConstantOutMin=[]  FilterDenConstantOutMax=[]  PCopyOutDataTypeStr=Inherit: Inherit via back propagation  PCopyOutMin=[]  PCopyOutMax=[]  NCopyOutDataTypeStr=Inherit: Inherit via back propagation  NCopyOutMin=[]  NCopyOutMax=[]  IntegratorContinuousStateAttributes=''  IntegratorStateMustResolveToSignalObject=off  IntegratorRTWStateStorageClass=Auto  FilterContinuousStateAttributes=''  FilterStateMustResolveToSignalObject=off  FilterRTWStateStorageClass=Auto  ParallelPVariant=InternalParameters  IdealPVariant=Disabled  IVariant=InternalParameters  DVariant=InternalParameters  IntegratorVariant=Continuous  SatVariant=Disabled  AWVariant=Passthrough  PCopyVariant=Disabled  TRVariant=Disabled  FdbkBlocksVariant=Forward  IdealPFdbkVariant=Disabled  SatFdbkVariant=Disabled  DerivativeFilterVariant=ContFilter  NVariant=InternalParameters  NCopyVariant=Disabled  FilterICVariant=InternalICsFilter  IntegratorICVariant=InternalICs  ExternalResetVariant=Disabled  TRSumVariant=Passthrough  SumFdbkVariant=Disabled  SumVariant=Sum_PID  TsampFilterVariant=InternalTs  TsampNgainVariant=Passthrough  TsampIntegralVariant=Disabled_SignalSpec  ExternalSaturationOutDataTypeStr=Inherit: Same as second input  DerivativeSourceVariant=ErrorSignal  PreIntVariant=InternalPreInt
  PID Controller2 : slpidlib/PID Controller  Controller=PID  Form=Parallel  TimeDomain=Continuous-time  UseExternalTs=off  SampleTime=-1  IntegratorMethod=Forward Euler  FilterMethod=Forward Euler  ControllerParametersSource=internal  P=0.207161142928572  I=0.156816263859124  UseKiTs=off  D=0.047326492099125  UseExternalDerivativeSource=off  N=21.4472408149846  UseFilter=on  TunerSelectOption=Transfer Function Based (PID Tuner App)  InitialConditionSource=internal  InitialConditionForIntegrator=0  InitialConditionForFilter=0  DifferentiatorICPrevScaledInput=0  ExternalReset=none  TrackingMode=off  Kt=1  LimitOutput=off  SatLimitsSource=internal  UpperSaturationLimit=inf  LowerSaturationLimit=-inf  LinearizeAsGain=on  AntiWindupMode=none  Kb=1  LimitIntegrator=off  UpperIntegratorSaturationLimit=inf  LowerIntegratorSaturationLimit=-inf  POutMin=[]  POutMax=[]  IOutMin=[]  IOutMax=[]  DOutMin=[]  DOutMax=[]  NOutMin=[]  NOutMax=[]  SumOutMin=[]  SumOutMax=[]  SaturationOutMin=[]  SaturationOutMax=[]  PParamMin=[]  PParamMax=[]  IParamMin=[]  IParamMax=[]  DParamMin=[]  DParamMax=[]  NParamMin=[]  NParamMax=[]  KbParamMin=[]  KbParamMax=[]  KtParamMin=[]  KtParamMax=[]  KbOutMin=[]  KbOutMax=[]  KtOutMin=[]  KtOutMax=[]  IntegratorOutMin=[]  IntegratorOutMax=[]  FilterOutMin=[]  FilterOutMax=[]  SumI1OutMin=[]  SumI1OutMax=[]  SumI2OutMin=[]  SumI2OutMax=[]  SumI3OutMin=[]  SumI3OutMax=[]  SumI4OutMin=[]  SumI4OutMax=[]  SumDOutMin=[]  SumDOutMax=[]  DifferentiatorOutMin=[]  DifferentiatorOutMax=[]  FilterDiffOutCoefMin=[]  FilterDiffOutCoefMax=[]  ReciprocalOutMin=[]  ReciprocalOutMax=[]  SumDenOutMin=[]  SumDenOutMax=[]  SumNumOutMin=[]  SumNumOutMax=[]  DivideOutMin=[]  DivideOutMax=[]  UdiffTsProdOutMin=[]  UdiffTsProdOutMax=[]  NTsProdOutMin=[]  NTsProdOutMax=[]  UintegralTsProdOutMin=[]  UintegralTsProdOutMax=[]  UngainTsProdOutMin=[]  UngainTsProdOutMax=[]  ClampingZeroOutDataTypeStr=Inherit: Inherit via back propagation  ClampingZeroOutMin=[]  ClampingZeroOutMax=[]  FilterDenConstantOutDataTypeStr=Inherit: Inherit via back propagation  FilterDenConstantOutMin=[]  FilterDenConstantOutMax=[]  PCopyOutDataTypeStr=Inherit: Inherit via back propagation  PCopyOutMin=[]  PCopyOutMax=[]  NCopyOutDataTypeStr=Inherit: Inherit via back propagation  NCopyOutMin=[]  NCopyOutMax=[]  IntegratorContinuousStateAttributes=''  IntegratorStateMustResolveToSignalObject=off  IntegratorRTWStateStorageClass=Auto  FilterContinuousStateAttributes=''  FilterStateMustResolveToSignalObject=off  FilterRTWStateStorageClass=Auto  ParallelPVariant=InternalParameters  IdealPVariant=Disabled  IVariant=InternalParameters  DVariant=InternalParameters  IntegratorVariant=Continuous  SatVariant=Disabled  AWVariant=Passthrough  PCopyVariant=Disabled  TRVariant=Disabled  FdbkBlocksVariant=Forward  IdealPFdbkVariant=Disabled  SatFdbkVariant=Disabled  DerivativeFilterVariant=ContFilter  NVariant=InternalParameters  NCopyVariant=Disabled  FilterICVariant=InternalICsFilter  IntegratorICVariant=InternalICs  ExternalResetVariant=Disabled  TRSumVariant=Passthrough  SumFdbkVariant=Disabled  SumVariant=Sum_PID  TsampFilterVariant=InternalTs  TsampNgainVariant=Passthrough  TsampIntegralVariant=Disabled_SignalSpec  ExternalSaturationOutDataTypeStr=Inherit: Same as second input  DerivativeSourceVariant=ErrorSignal  PreIntVariant=InternalPreInt
  PID Controller3 : slpidlib/PID Controller  Controller=PID  Form=Parallel  TimeDomain=Continuous-time  UseExternalTs=off  SampleTime=-1  IntegratorMethod=Forward Euler  FilterMethod=Forward Euler  ControllerParametersSource=internal  P=2.11820553187522  I=4.01210446281075  UseKiTs=off  D=0.16220869399402  UseExternalDerivativeSource=off  N=87.1466857594837  UseFilter=on  TunerSelectOption=Transfer Function Based (PID Tuner App)  InitialConditionSource=internal  InitialConditionForIntegrator=0  InitialConditionForFilter=0  DifferentiatorICPrevScaledInput=0  ExternalReset=none  TrackingMode=off  Kt=1  LimitOutput=off  SatLimitsSource=internal  UpperSaturationLimit=inf  LowerSaturationLimit=-inf  LinearizeAsGain=on  AntiWindupMode=none  Kb=1  LimitIntegrator=off  UpperIntegratorSaturationLimit=inf  LowerIntegratorSaturationLimit=-inf  POutMin=[]  POutMax=[]  IOutMin=[]  IOutMax=[]  DOutMin=[]  DOutMax=[]  NOutMin=[]  NOutMax=[]  SumOutMin=[]  SumOutMax=[]  SaturationOutMin=[]  SaturationOutMax=[]  PParamMin=[]  PParamMax=[]  IParamMin=[]  IParamMax=[]  DParamMin=[]  DParamMax=[]  NParamMin=[]  NParamMax=[]  KbParamMin=[]  KbParamMax=[]  KtParamMin=[]  KtParamMax=[]  KbOutMin=[]  KbOutMax=[]  KtOutMin=[]  KtOutMax=[]  IntegratorOutMin=[]  IntegratorOutMax=[]  FilterOutMin=[]  FilterOutMax=[]  SumI1OutMin=[]  SumI1OutMax=[]  SumI2OutMin=[]  SumI2OutMax=[]  SumI3OutMin=[]  SumI3OutMax=[]  SumI4OutMin=[]  SumI4OutMax=[]  SumDOutMin=[]  SumDOutMax=[]  DifferentiatorOutMin=[]  DifferentiatorOutMax=[]  FilterDiffOutCoefMin=[]  FilterDiffOutCoefMax=[]  ReciprocalOutMin=[]  ReciprocalOutMax=[]  SumDenOutMin=[]  SumDenOutMax=[]  SumNumOutMin=[]  SumNumOutMax=[]  DivideOutMin=[]  DivideOutMax=[]  UdiffTsProdOutMin=[]  UdiffTsProdOutMax=[]  NTsProdOutMin=[]  NTsProdOutMax=[]  UintegralTsProdOutMin=[]  UintegralTsProdOutMax=[]  UngainTsProdOutMin=[]  UngainTsProdOutMax=[]  ClampingZeroOutDataTypeStr=Inherit: Inherit via back propagation  ClampingZeroOutMin=[]  ClampingZeroOutMax=[]  FilterDenConstantOutDataTypeStr=Inherit: Inherit via back propagation  FilterDenConstantOutMin=[]  FilterDenConstantOutMax=[]  PCopyOutDataTypeStr=Inherit: Inherit via back propagation  PCopyOutMin=[]  PCopyOutMax=[]  NCopyOutDataTypeStr=Inherit: Inherit via back propagation  NCopyOutMin=[]  NCopyOutMax=[]  IntegratorContinuousStateAttributes=''  IntegratorStateMustResolveToSignalObject=off  IntegratorRTWStateStorageClass=Auto  FilterContinuousStateAttributes=''  FilterStateMustResolveToSignalObject=off  FilterRTWStateStorageClass=Auto  ParallelPVariant=InternalParameters  IdealPVariant=Disabled  IVariant=InternalParameters  DVariant=InternalParameters  IntegratorVariant=Continuous  SatVariant=Disabled  AWVariant=Passthrough  PCopyVariant=Disabled  TRVariant=Disabled  FdbkBlocksVariant=Forward  IdealPFdbkVariant=Disabled  SatFdbkVariant=Disabled  DerivativeFilterVariant=ContFilter  NVariant=InternalParameters  NCopyVariant=Disabled  FilterICVariant=InternalICsFilter  IntegratorICVariant=InternalICs  ExternalResetVariant=Disabled  TRSumVariant=Passthrough  SumFdbkVariant=Disabled  SumVariant=Sum_PID  TsampFilterVariant=InternalTs  TsampNgainVariant=Passthrough  TsampIntegralVariant=Disabled_SignalSpec  ExternalSaturationOutDataTypeStr=Inherit: Same as second input  DerivativeSourceVariant=ErrorSignal  PreIntVariant=InternalPreInt
  Scope : Scope  NumInputPorts=4
  Sum{,1..3} (4 alike) : Sum  Inputs=|+-
  Sum4 : Sum  Inputs=++|
  Terminator : Terminator
  Terminator1 : Terminator
  Thrust(t) : Scope
  gravity pre-compensation : Constant  Value=m*g
  Fz,mx,my,mz : Outport
  wires:
  Mux/1 -> Fz,mx,my,mz/1
  Sum/1 -> PID Controller/1
  Demux/2 -> Degrees to Radians/1
  Demux/3 -> Degrees to Radians1/1
  Demux/4 -> Degrees to Radians2/1
  desired z,phictheta,psi/1 -> Demux/1
  eta/1 -> Demux1/1
  Demux1/1 -> Terminator/1
  Demux1/4 -> Sum1/2
  Demux1/5 -> Sum2/2
  Demux1/6 -> Sum3/2
  Degrees to Radians/1 -> Sum1/1
  Degrees to Radians1/1 -> Sum2/1
  Degrees to Radians2/1 -> Sum3/1
  Demux/1 -> Sum/1
  PID Controller/1 -> Sum4/2
  gravity pre-compensation/1 -> Sum4/1
  Demux1/2 -> Terminator1/1
  Demux1/3 -> Sum/2
  Sum4/1 -> Thrust(t)/1, Mux/1, Scope/1
  Sum1/1 -> PID Controller1/1
  Sum2/1 -> PID Controller2/1
  Sum3/1 -> PID Controller3/1
  PID Controller1/1 -> Mux/2, Scope/2
  PID Controller2/1 -> Mux/3, Scope/3
  PID Controller3/1 -> Mux/4, Scope/4

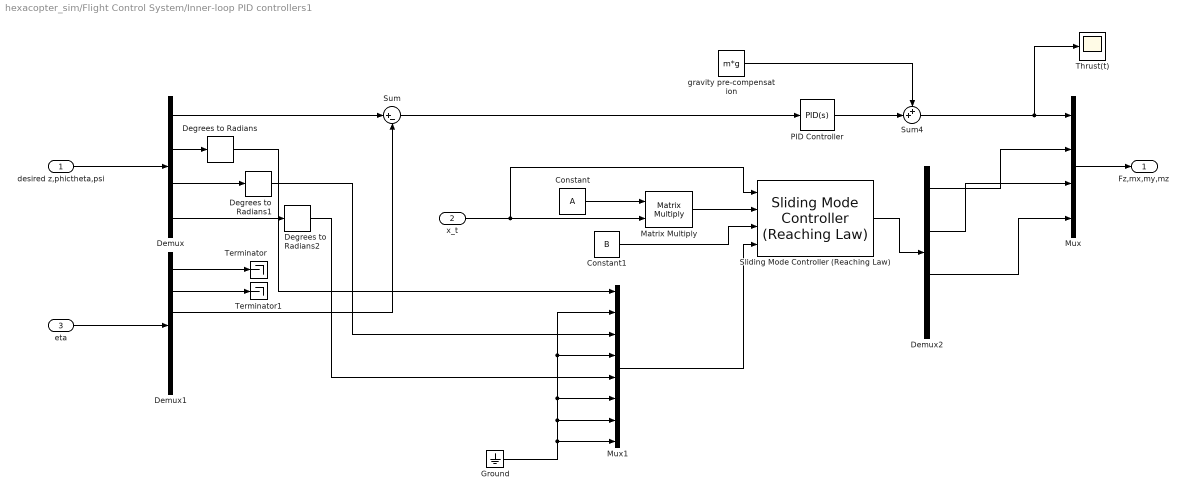
== system hexacopter_sim/Flight Control System/Inner-loop PID controllers1 ==
  desired z,phictheta,psi : Inport
  x_t : Inport  Port=2
  eta : Inport  Port=3
  Constant : Constant  Value=A
  Constant1 : Constant  Value=B
  Degrees to Radians : simulink_extras/Transformations/Degrees to Radians
  Degrees to Radians1 : simulink_extras/Transformations/Degrees to Radians
  Degrees to Radians2 : simulink_extras/Transformations/Degrees to Radians
  Demux : Demux
  Demux1 : Demux  Outputs=6
  Demux2 : Demux
  Ground : Ground
  Matrix Multiply : Product  Multiplication=Matrix(*)
  Mux : Mux
  Mux1 : Mux  Inputs=8
  PID Controller : slpidlib/PID Controller  Controller=PID  Form=Parallel  TimeDomain=Continuous-time  UseExternalTs=off  SampleTime=-1  IntegratorMethod=Forward Euler  FilterMethod=Forward Euler  ControllerParametersSource=internal  P=174437.007400364  I=18036.2798671007  UseKiTs=off  D=411426.319993485  UseExternalDerivativeSource=off  N=10.9079405084324  UseFilter=on  TunerSelectOption=Transfer Function Based (PID Tuner App)  InitialConditionSource=internal  InitialConditionForIntegrator=0  InitialConditionForFilter=0  DifferentiatorICPrevScaledInput=0  ExternalReset=none  TrackingMode=off  Kt=1  LimitOutput=off  SatLimitsSource=internal  UpperSaturationLimit=inf  LowerSaturationLimit=-inf  LinearizeAsGain=on  AntiWindupMode=none  Kb=1  LimitIntegrator=off  UpperIntegratorSaturationLimit=inf  LowerIntegratorSaturationLimit=-inf  POutMin=[]  POutMax=[]  IOutMin=[]  IOutMax=[]  DOutMin=[]  DOutMax=[]  NOutMin=[]  NOutMax=[]  SumOutMin=[]  SumOutMax=[]  SaturationOutMin=[]  SaturationOutMax=[]  PParamMin=[]  PParamMax=[]  IParamMin=[]  IParamMax=[]  DParamMin=[]  DParamMax=[]  NParamMin=[]  NParamMax=[]  KbParamMin=[]  KbParamMax=[]  KtParamMin=[]  KtParamMax=[]  KbOutMin=[]  KbOutMax=[]  KtOutMin=[]  KtOutMax=[]  IntegratorOutMin=[]  IntegratorOutMax=[]  FilterOutMin=[]  FilterOutMax=[]  SumI1OutMin=[]  SumI1OutMax=[]  SumI2OutMin=[]  SumI2OutMax=[]  SumI3OutMin=[]  SumI3OutMax=[]  SumI4OutMin=[]  SumI4OutMax=[]  SumDOutMin=[]  SumDOutMax=[]  DifferentiatorOutMin=[]  DifferentiatorOutMax=[]  FilterDiffOutCoefMin=[]  FilterDiffOutCoefMax=[]  ReciprocalOutMin=[]  ReciprocalOutMax=[]  SumDenOutMin=[]  SumDenOutMax=[]  SumNumOutMin=[]  SumNumOutMax=[]  DivideOutMin=[]  DivideOutMax=[]  UdiffTsProdOutMin=[]  UdiffTsProdOutMax=[]  NTsProdOutMin=[]  NTsProdOutMax=[]  UintegralTsProdOutMin=[]  UintegralTsProdOutMax=[]  UngainTsProdOutMin=[]  UngainTsProdOutMax=[]  ClampingZeroOutDataTypeStr=Inherit: Inherit via back propagation  ClampingZeroOutMin=[]  ClampingZeroOutMax=[]  FilterDenConstantOutDataTypeStr=Inherit: Inherit via back propagation  FilterDenConstantOutMin=[]  FilterDenConstantOutMax=[]  PCopyOutDataTypeStr=Inherit: Inherit via back propagation  PCopyOutMin=[]  PCopyOutMax=[]  NCopyOutDataTypeStr=Inherit: Inherit via back propagation  NCopyOutMin=[]  NCopyOutMax=[]  IntegratorContinuousStateAttributes=''  IntegratorStateMustResolveToSignalObject=off  IntegratorRTWStateStorageClass=Auto  FilterContinuousStateAttributes=''  FilterStateMustResolveToSignalObject=off  FilterRTWStateStorageClass=Auto  ParallelPVariant=InternalParameters  IdealPVariant=Disabled  IVariant=InternalParameters  DVariant=InternalParameters  IntegratorVariant=Continuous  SatVariant=Disabled  AWVariant=Passthrough  PCopyVariant=Disabled  TRVariant=Disabled  FdbkBlocksVariant=Forward  IdealPFdbkVariant=Disabled  SatFdbkVariant=Disabled  DerivativeFilterVariant=ContFilter  NVariant=InternalParameters  NCopyVariant=Disabled  FilterICVariant=InternalICsFilter  IntegratorICVariant=InternalICs  ExternalResetVariant=Disabled  TRSumVariant=Passthrough  SumFdbkVariant=Disabled  SumVariant=Sum_PID  TsampFilterVariant=InternalTs  TsampNgainVariant=Passthrough  TsampIntegralVariant=Disabled_SignalSpec  ExternalSaturationOutDataTypeStr=Inherit: Same as second input  DerivativeSourceVariant=ErrorSignal  PreIntVariant=InternalPreInt
  Sliding Mode Controller (Reaching Law) : slctrl_smc/Sliding Mode Controller (Reaching Law)  TaskMode=Tracking Mode  SlidingMatrix=C_ls  EnableTrackingDerivative=off  EnableSwitchingFunction=off  ReachingLaw=Constant Rate  ReachingRate=0.01  ControlGain=0.01  PowerRate=0.01  BoundaryLayer=Sign  Phi=0.01
  Sum : Sum  Inputs=|+-
  Sum4 : Sum  Inputs=++|
  Terminator : Terminator
  Terminator1 : Terminator
  Thrust(t) : Scope
  gravity pre-compensation : Constant  Value=m*g
  Fz,mx,my,mz : Outport
  wires:
  PID Controller/1 -> Sum4/2
  Demux/1 -> Sum/1
  Demux/2 -> Degrees to Radians/1
  Mux/1 -> Fz,mx,my,mz/1
  Demux1/2 -> Terminator1/1
  Demux1/3 -> Sum/2
  Demux/3 -> Degrees to Radians1/1
  Demux/4 -> Degrees to Radians2/1
  Sum4/1 -> Thrust(t)/1, Mux/1
  eta/1 -> Demux1/1
  Sum/1 -> PID Controller/1
  gravity pre-compensation/1 -> Sum4/1
  Demux1/1 -> Terminator/1
  desired z,phictheta,psi/1 -> Demux/1
  Matrix Multiply/1 -> Sliding Mode Controller (Reaching Law)/2
  x_t/1 -> Sliding Mode Controller (Reaching Law)/1, Matrix Multiply/2
  Constant/1 -> Matrix Multiply/1
  Constant1/1 -> Sliding Mode Controller (Reaching Law)/3
  Degrees to Radians/1 -> Mux1/1
  Degrees to Radians1/1 -> Mux1/3
  Degrees to Radians2/1 -> Mux1/5
  Mux1/1 -> Sliding Mode Controller (Reaching Law)/4
  Ground/1 -> Mux1/8, Mux1/7, Mux1/4, Mux1/2, Mux1/6
  Sliding Mode Controller (Reaching Law)/1 -> Demux2/1
  Demux2/1 -> Mux/2
  Demux2/2 -> Mux/3
  Demux2/3 -> Mux/4
